simulink model "fallschirmTransferBlock"  (R2018b)
settings: Solver=ode45  StartTime=0.0  StopTime=inf  RelTol=1e-3  EnableMultiTasking=on
model workspace (MAT data in the model file):
  AFS = 30
  AS = 0.5
  cw = 1.3
  g = 9.81
  h0 = 500
  h1 = 20
  m = 85
  rho = 1.2
  v0 = 0
settings Model: Creator=Reichl  LastModifiedBy=Reichl
settings DataIOCC: SaveFormat=Array  OutputSaveName=h
settings OptimizationCC: LifeSpan=inf
settings DebuggingCC: SolverPrmCheckMsg=warning  AllowSymbolicDim=off  SFUnexpectedBacktrackingDiag=warning  SFNoUnconditionalDefaultTransitionDiag=warning  SFExecutionAtInitializationDiag=none
settings HardwareCC: ProdBitPerPointer=32  ProdBitPerSizeT=32  ProdBitPerPtrDiffT=32  ProdLargestAtomicFloat=None  ProdIntDivRoundTo=Undefined  ProdEndianess=Unspecified  ProdWordSize=32  ProdHWDeviceType=32-bit Generic
settings ModelReferenceCC: PropagateSignalLabelsOutOfModel=off
settings SFSimCC: SimUseLocalCustomCode=off
settings RTWCC: RTWUseLocalCustomCode=off
settings CodeAppCC: StateflowObjectComments=on
settings GRTTargetCC: TargetLangStandard=C89/C90 (ANSI)  GeneratePreprocessorConditionals=Disable all
settings ConfigComp: CovMetricSettings=dw  CovHtmlReporting=on  CovSaveCumulativeToWorkspaceVar=on  CovSaveSingleToWorkspaceVar=on  CovExternalEMLEnable=off  CovSFcnEnable=off

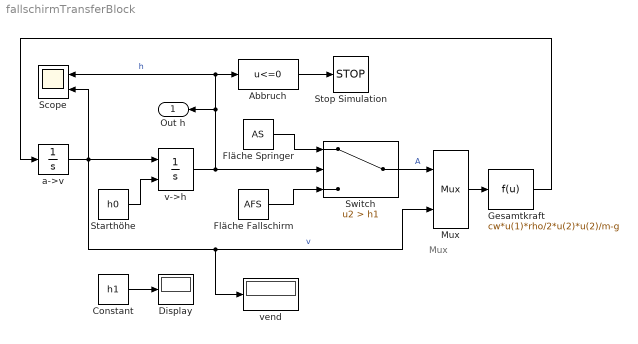
== system fallschirmTransferBlock ==
  note: Mux
  Abbruch : Fcn  Expr=u<=0
  Constant : Constant  Value=h1
  Display : Display
  Fläche Fallschirm : Constant  Value=AFS
  Fläche Springer : Constant  Value=AS
  Gesamtkraft : Fcn  Expr=cw*u(1)*rho/2*u(2)*u(2)/m-g
  Mux : Mux  Inputs=2
      settings: DisplayOption=signals
  Scope : Scope  NumInputPorts=2
  Starthöhe : Constant  Value=h0
  Stop Simulation : Stop
  Switch : Switch  Criteria=u2 > Threshold  Threshold=h1  ZeroCross=off
  a->v : Integrator  InitialCondition=v0
  v->h : Integrator  InitialConditionSource=external
  vend : Display
  Out h : Outport
  wires:
  a->v/1 -> vend/1, Mux/2, Scope/2, v->h/1  "v"
  v->h/1 -> Out h/1, Scope/1, Abbruch/1, Switch/2  "h"
  Fläche Springer/1 -> Switch/1
  Fläche Fallschirm/1 -> Switch/3
  Switch/1 -> Mux/1  "A"
  Abbruch/1 -> Stop Simulation/1
  Starthöhe/1 -> v->h/2
  Mux/1 -> Gesamtkraft/1
  Gesamtkraft/1 -> a->v/1
  Constant/1 -> Display/1
